simulink model "viterby4"  (R2022b)
settings: Solver=FixedStepAuto  StartTime=0.0  StopTime=10  FixedStep=0.1  RelTol=1e-3
libraries: simulink_extras x5, simulink x2, hdlsllib x1
settings Model: Creator=user  LastModifiedBy=Karolina
settings SolverCC: AlgebraicLoopSolver=TrustRegion
settings DebuggingCC: UnconnectedInputMsg=warning  UnconnectedOutputMsg=warning  UnconnectedLineMsg=warning  SFMachineParentedDataDiag=warning
settings ModelReferenceCC: EnableRefExpFcnMdlSchedulingChecks=on
settings SFSimCC: CustomCodeUndefinedFunction=UseInterfaceOnly
settings RTWCC: DLArmComputeVersion=19.05

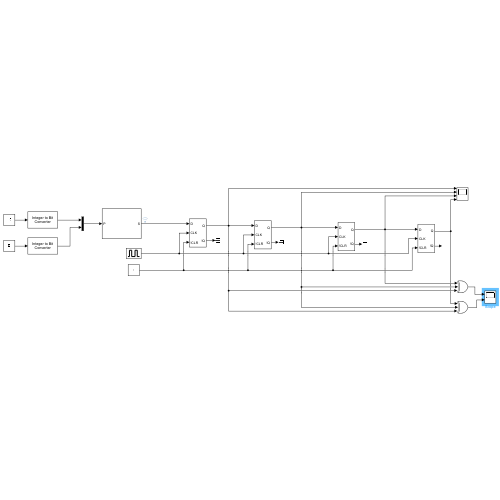
[thumbnail: Simulink's stored preview of the top-level diagram]
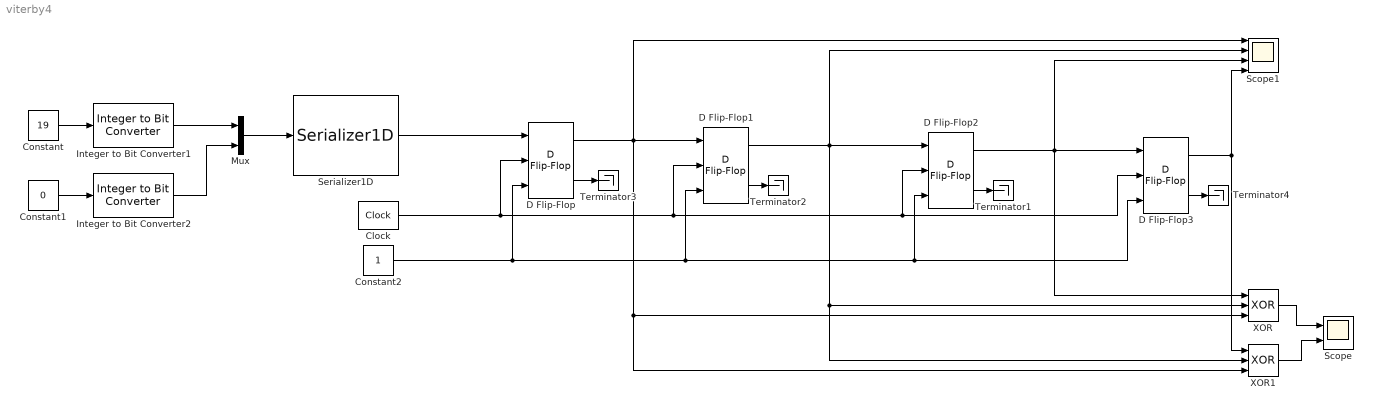
== system viterby4 ==
  Clock : simulink_extras/Flip Flops/Clock  period=1
  Constant : Constant  Value=19
  Constant1 : Constant  Value=0
  Constant2 : Constant  OutDataTypeStr=boolean
  D Flip-Flop{,1..3} (4 alike) : simulink_extras/Flip Flops/D Flip-Flop
  Integer to Bit Converter1 : simulink/Logic and Bit Operations/Integer to Bit Converter  nbits=5  signedInputValues=Unsigned  bitOrder=MSB first  outDtype=boolean
      settings: LibrarySourceBlock=|
      | commutil2/Integer to Bit
      | Converter
  Integer to Bit Converter2 : simulink/Logic and Bit Operations/Integer to Bit Converter  nbits=4  signedInputValues=Unsigned  bitOrder=MSB first  outDtype=boolean
      settings: LibrarySourceBlock=|
      | commutil2/Integer to Bit
      | Converter
  Mux : Mux  Inputs=2
  Scope : Scope  NumInputPorts=2
  Scope1 : Scope  NumInputPorts=4
  Serializer1D : hdlsllib/HDL Operations/Serializer1D  Ratio=9  IdleCycles=0  validIn=off  startOut=off  validOut=off  inputDataDimensions=-1  inputSampleTime=9  inputSignalType=auto
  Terminator{1..4} (4 alike) : Terminator
  XOR : Logic  Operator=XOR  Inputs=3  IconShape=distinctive  AllPortsSameDT=off  OutDataTypeStr=boolean
  XOR1 : Logic  Operator=XOR  Inputs=3  IconShape=distinctive  AllPortsSameDT=off  OutDataTypeStr=boolean
  wires:
  Constant/1 -> Integer to Bit Converter1/1
  Serializer1D/1 -> D Flip-Flop/1
  D Flip-Flop1/1 -> XOR1/2, XOR/2, Scope1/2, D Flip-Flop2/1
  D Flip-Flop/1 -> Scope1/1, D Flip-Flop1/1, XOR1/3, XOR/3
  D Flip-Flop2/2 -> Terminator1/1
  D Flip-Flop1/2 -> Terminator2/1
  D Flip-Flop/2 -> Terminator3/1
  Clock/1 -> D Flip-Flop/2, D Flip-Flop1/2, D Flip-Flop2/2, D Flip-Flop3/2
  D Flip-Flop3/2 -> Terminator4/1
  Constant2/1 -> D Flip-Flop/3, D Flip-Flop1/3, D Flip-Flop2/3, D Flip-Flop3/3
  D Flip-Flop2/1 -> XOR/1, D Flip-Flop3/1, Scope1/3
  D Flip-Flop3/1 -> Scope1/4, XOR1/1
  XOR/1 -> Scope/1
  XOR1/1 -> Scope/2
  Mux/1 -> Serializer1D/1
  Integer to Bit Converter1/1 -> Mux/1
  Constant1/1 -> Integer to Bit Converter2/1
  Integer to Bit Converter2/1 -> Mux/2
